simulink model "pendoloSim"  (R2020a)
settings: Solver=VariableStepAuto  StartTime=0.0  StopTime=100.0  RelTol=1e-3
values from neighbouring files (symbols this model uses):
  Fr = 4    [pendolo.m]    (also in pendolo2.m; pendoloGlobal.m)
  g = 9.81    [pendolo.m]    (also in pendolo2.m = 9.8; pendoloGlobal.m)
  l = 0.2    [generatrice.m]    (also in pendolo.m = 5; pendolo2.m = 5; pendoloGlobal.m = 5)
  m = 0.5    [generatrice.m]    (also in pendolo.m = 30; pendolo2.m = 30; pendoloGlobal.m = 30)
settings Model: Creator=aless  LastModifiedBy=aless

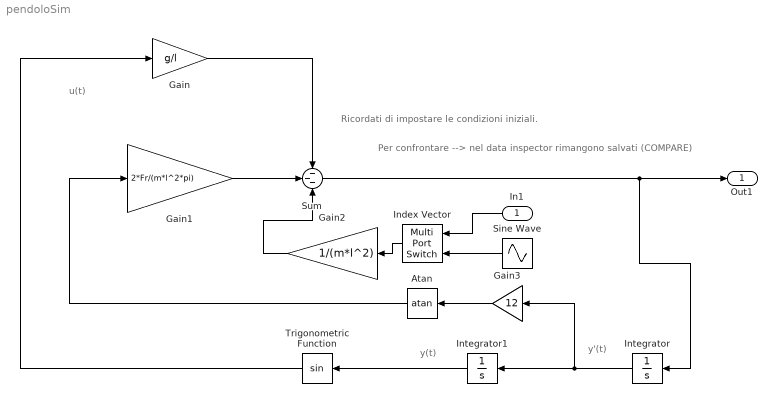
== system pendoloSim ==
  note: Per confrontare --> nel data inspector rimangono salvati (COMPARE)
  note: Ricordati di impostare le condizioni iniziali.
  note: y(t)
  note: y'(t)
  note: u(t)
  In1 : Inport
  Atan : Trigonometry  Operator=atan
  Gain : Gain  Gain=g/l
  Gain1 : Gain  Gain=2*Fr/(m*l^2*pi)
  Gain2 : Gain  Gain=1/(m*l^2)
  Gain3 : Gain  Gain=12
  Index Vector : MultiPortSwitch  DataPortOrder=Zero-based contiguous  Inputs=1  zeroidx=on
  Integrator : Integrator
  Integrator1 : Integrator  InitialCondition=1/2
  Sine Wave : Sin  Amplitude=30  Frequency=2*pi*0.1  SampleTime=0
  Sum : Sum  Inputs=---
  Trigonometric Function : Trigonometry
  Out1 : Outport
  wires:
  Gain1/1 -> Sum/2
  Gain/1 -> Sum/1
  Gain2/1 -> Sum/3
  Sum/1 -> Integrator/1, Out1/1
  Integrator/1 -> Gain3/1, Integrator1/1
  Integrator1/1 -> Trigonometric Function/1
  Trigonometric Function/1 -> Gain/1
  Gain3/1 -> Atan/1
  Atan/1 -> Gain1/1
  Index Vector/1 -> Gain2/1
  In1/1 -> Index Vector/1
  Sine Wave/1 -> Index Vector/2
